simulink model "Base"  (R2023b)
settings: Solver=ode3  StartTime=0.0  StopTime=inf  RelTol=1e-3  EnableMultiTasking=on
libraries: arduinolib x4, simulink x3, arduinosensorlib x3
settings Model: FPTRunName=Active  ExtModeTrigDuration=2  Creator=SCBR-HP  LastModifiedBy=Rafael
settings SolverCC: AlgebraicLoopSolver=TrustRegion
settings DataIOCC: LimitDataPoints=on  SaveFormat=Array
settings OptimizationCC: ReuseModelBlockBuffer=off  ExpressionDepthLimit=2147483647  LifeSpan=Inf  MaxStackSize=64
settings DebuggingCC: UnderspecifiedInitializationDetection=Classic  MergeDetectMultiDrivingBlocksExec=none  FcnCallInpInsideContextMsg=warning  UnconnectedInputMsg=warning  UnconnectedOutputMsg=warning  UnconnectedLineMsg=warning  AllowSymbolicDim=off  StateNameClashWarn=warning  SFUnexpectedBacktrackingDiag=warning  SFNoUnconditionalDefaultTransitionDiag=warning  SFExecutionAtInitializationDiag=none  ArithmeticOperatorsInVariantConditions=warning
settings HardwareCC: ProdBitPerPointer=32  ProdBitPerSizeT=32  ProdBitPerPtrDiffT=32  ProdLargestAtomicInteger=Long  ProdLargestAtomicFloat=Double  ProdWordSize=32  ProdHWDeviceType=ARM Compatible->ARM Cortex  UseEmbeddedCoderFeatures=off  UseSimulinkCoderFeatures=off
settings ModelReferenceCC: EnableRefExpFcnMdlSchedulingChecks=on  PropagateSignalLabelsOutOfModel=off
settings SFSimCC: SimUseLocalCustomCode=off  CustomCodeUndefinedFunction=UseInterfaceOnly
settings RTWCC: Description=Embedded Coder  SystemTargetFile=ert.tlc  HardwareBoard=Arduino Due  TemplateMakefile=ert_default_tmf  GenerateReport=on  RTWVerbose=off  RTWUseLocalCustomCode=off  Toolchain=Arduino ARM  BuildConfiguration=Faster Runs  LaunchReport=on
settings CodeAppCC: ForceParamTrailComments=on  OperatorAnnotations=on  MangleLength=10  StateflowObjectComments=on  MATLABSourceComments=on
settings ERTTargetCC: MultiwordLength=2048  ERTCustomFileBanners=off  SupportContinuousTime=on  SupportNonInlinedSFcns=on  RemoveResetFunc=off  SupportVariableSizeSignals=on  ModelStepFunctionPrototypeControlCompliant=off  ExtModeTransport=3  ExtModeStaticAlloc=on  ExtModeAutomaticAllocSize=off  ExtModeStaticAllocSize=24576  ExtModeMexFile=ext_xcp  ExtModeIntrfLevel=Level2 - Open
settings ConfigComp: CovMetricSettings=dw  CovSaveCumulativeToWorkspaceVar=on  CovSaveSingleToWorkspaceVar=on  CovExternalEMLEnable=off  CovSFcnEnable=off

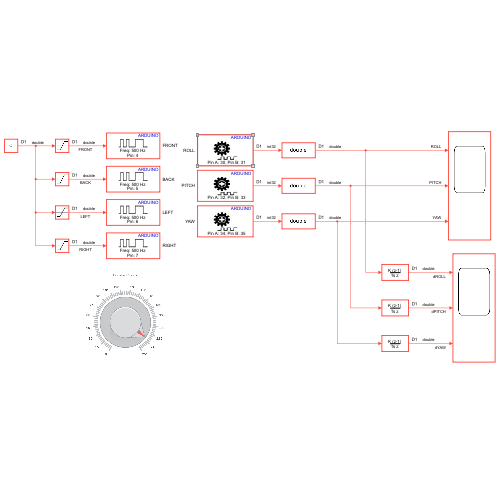
[thumbnail: Simulink's stored preview of the top-level diagram]
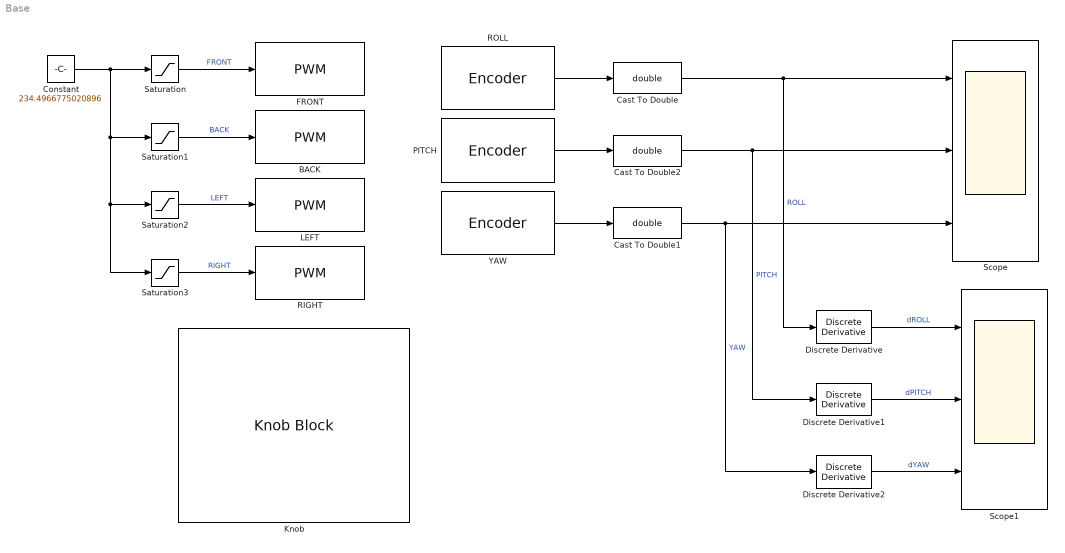
== system Base ==
  BACK : arduinolib/PWM  pinNumber=5  frequencyType=Specify  desiredFrequency=500  achievableFrequency=500
  Cast To Double : DataTypeConversion  OutDataTypeStr=double  SaturateOnIntegerOverflow=off  RndMeth=Floor
  Cast To Double1 : DataTypeConversion  OutDataTypeStr=double  SaturateOnIntegerOverflow=off  RndMeth=Floor
  Cast To Double2 : DataTypeConversion  OutDataTypeStr=double  SaturateOnIntegerOverflow=off  RndMeth=Floor
  Constant : Constant  Value=234.4966775020896  SampleTime=1/50
  Discrete Derivative : simulink/Discrete/Discrete Derivative  gainval=1.0  ICPrevScaledInput=0.0  OutMin=[]  OutMax=[]  OutDataType=fixdt(1, 16)  OutScaling=2^-10  DoSatur=off
  Discrete Derivative1 : simulink/Discrete/Discrete Derivative  gainval=1.0  ICPrevScaledInput=0.0  OutMin=[]  OutMax=[]  OutDataType=fixdt(1, 16)  OutScaling=2^-10  DoSatur=off
  Discrete Derivative2 : simulink/Discrete/Discrete Derivative  gainval=1.0  ICPrevScaledInput=0.0  OutMin=[]  OutMax=[]  OutDataType=fixdt(1, 16)  OutScaling=2^-10  DoSatur=off
  FRONT : arduinolib/PWM  pinNumber=4  frequencyType=Specify  desiredFrequency=500  achievableFrequency=500
  Knob : KnobBlock  ScaleMax=255
  LEFT : arduinolib/PWM  pinNumber=6  frequencyType=Specify  desiredFrequency=500  achievableFrequency=500
  PITCH : arduinosensorlib/Encoder  InputA=32  InputB=33  Mode=No reset  SampleTime=1/50
  RIGHT : arduinolib/PWM  pinNumber=7  frequencyType=Specify  desiredFrequency=500  achievableFrequency=500
  ROLL : arduinosensorlib/Encoder  InputA=30  InputB=31  Mode=No reset  SampleTime=1/50
  Saturation{,1..3} (4 alike) : Saturate  UpperLimit=255  LowerLimit=0
  Scope : Scope  NumInputPorts=3
  Scope1 : Scope  NumInputPorts=3
  YAW : arduinosensorlib/Encoder  InputA=34  InputB=35  Mode=No reset  SampleTime=1/50
  wires:
  ROLL/1 -> Cast To Double/1
  PITCH/1 -> Cast To Double2/1
  Discrete Derivative/1 -> Scope1/1  "dROLL"
  Discrete Derivative1/1 -> Scope1/2  "dPITCH"
  Discrete Derivative2/1 -> Scope1/3  "dYAW"
  YAW/1 -> Cast To Double1/1
  Saturation/1 -> FRONT/1  "FRONT"
  Saturation1/1 -> BACK/1  "BACK"
  Saturation2/1 -> LEFT/1  "LEFT"
  Saturation3/1 -> RIGHT/1  "RIGHT"
  Cast To Double/1 -> Discrete Derivative/1, Scope/1  "ROLL"
  Cast To Double1/1 -> Scope/3, Discrete Derivative2/1  "YAW"
  Cast To Double2/1 -> Discrete Derivative1/1, Scope/2  "PITCH"
  Constant/1 -> Saturation3/1, Saturation2/1, Saturation1/1, Saturation/1
